simulink model "sensor_vehicle_modell"  (R2021a)
settings: Solver=ode3  StartTime=0.0  StopTime=70  FixedStep=0.01  RelTol=1e-3
values from neighbouring files (symbols this model uses):
  A = 2    [Parameter.m]
  cw = 0.0    (= 0)    [Parameter.m]
  d = 0.63    [Parameter.m]
  m = 1500    [Parameter.m]
  p = 1.2    [Parameter.m]
undefined symbols (not defined in the file or in its folder): DiscIntNeverNeededParam
libraries: simulink x4, simulink_extras x1
settings Model: Creator=ge78kon  LastModifiedBy=admin
settings SolverCC: AlgebraicLoopSolver=TrustRegion
settings DataIOCC: ReturnWorkspaceOutputs=off
settings DebuggingCC: SFMachineParentedDataDiag=warning  ArithmeticOperatorsInVariantConditions=warning
settings SFSimCC: CustomCodeUndefinedFunction=UseInterfaceOnly

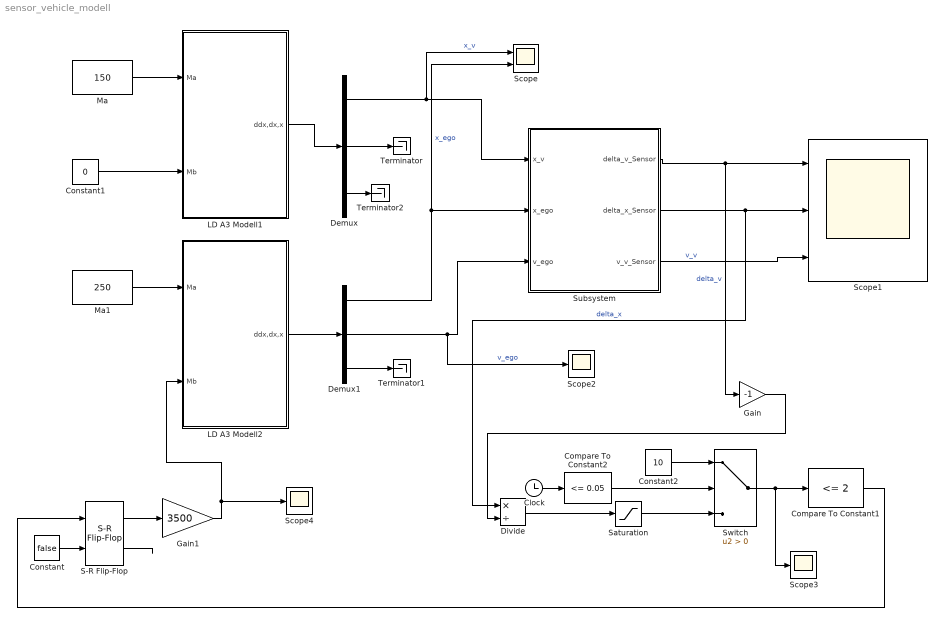
== system sensor_vehicle_modell ==
  Clock : Clock
  Compare To Constant1 : simulink/Logic and Bit Operations/Compare To Constant  relop=<=  const=2  OutDataTypeStr=boolean
  Compare To Constant2 : simulink/Logic and Bit Operations/Compare To Constant  relop=<=  const=0.05  OutDataTypeStr=boolean
  Constant : Constant  Value=false
  Constant1 : Constant  Value=0
  Constant2 : Constant  Value=10
  Demux : Demux  Outputs=3
  Demux1 : Demux  Outputs=3
  Divide : Product  Inputs=*/
  Gain : Gain  Gain=-1
  Gain1 : Gain  Gain=3500
  LD A3 Modell1 : Subsystem  mask{x_start=450, v_start=20}
      mask prompts: x_start "Startposition"; v_start "Startgeschwindigkeit"
  LD A3 Modell2 : Subsystem  mask{x_start=0, v_start=30}
      mask prompts: x_start "Startposition"; v_start "Startgeschwindigkeit"
  Ma : Constant  Value=150
  Ma1 : Constant  Value=250
  S-R Flip-Flop : simulink_extras/Flip Flops/S-R Flip-Flop  initial_condition=0
  Saturation : Saturate  UpperLimit=10
  Scope : Scope  NumInputPorts=2
  Scope1 : Scope  NumInputPorts=3
  Scope2 : Scope
  Scope3 : Scope
  Scope4 : Scope
  Subsystem : Subsystem  mask{Rauschen=off}
      mask prompts: Rauschen "Rauschen an/aus"
  Switch : Switch  Criteria=u2 > Threshold
  Terminator : Terminator
  Terminator1 : Terminator
  Terminator2 : Terminator
  wires:
  Ma/1 -> LD A3 Modell1/1("Ma ")
  Constant1/1 -> LD A3 Modell1/2("Mb ")
  LD A3 Modell1/1(ddx,dx,x) -> Demux/1
  LD A3 Modell2/1(ddx,dx,x) -> Demux1/1
  Ma1/1 -> LD A3 Modell2/1("Ma ")
  Demux/2 -> Terminator/1
  Demux1/3 -> Terminator1/1
  Demux/1 -> Scope/1, Subsystem/1(x_v)  "x_v"
  Demux1/1 -> Scope/2, Subsystem/2(x_ego)  "x_ego"
  Demux1/2 -> Scope2/1, Subsystem/3(v_ego)  "v_ego"
  Subsystem/1(delta_v_Sensor) -> Scope1/1, Gain/1  "delta_v"
  Subsystem/2(delta_x_Sensor) -> Divide/1, Scope1/2  "delta_x"
  Subsystem/3(v_v_Sensor) -> Scope1/3  "v_v"
  Demux/3 -> Terminator2/1
  Gain/1 -> Divide/2
  Divide/1 -> Saturation/1
  Compare To Constant1/1 -> S-R Flip-Flop/1
  S-R Flip-Flop/1 -> Gain1/1
  Gain1/1 -> LD A3 Modell2/2("Mb "), Scope4/1
  Constant/1 -> S-R Flip-Flop/2
  Clock/1 -> Compare To Constant2/1
  Compare To Constant2/1 -> Switch/2
  Constant2/1 -> Switch/1
  Saturation/1 -> Switch/3
  Switch/1 -> Scope3/1, Compare To Constant1/1
  S-R Flip-Flop/2 -> ?

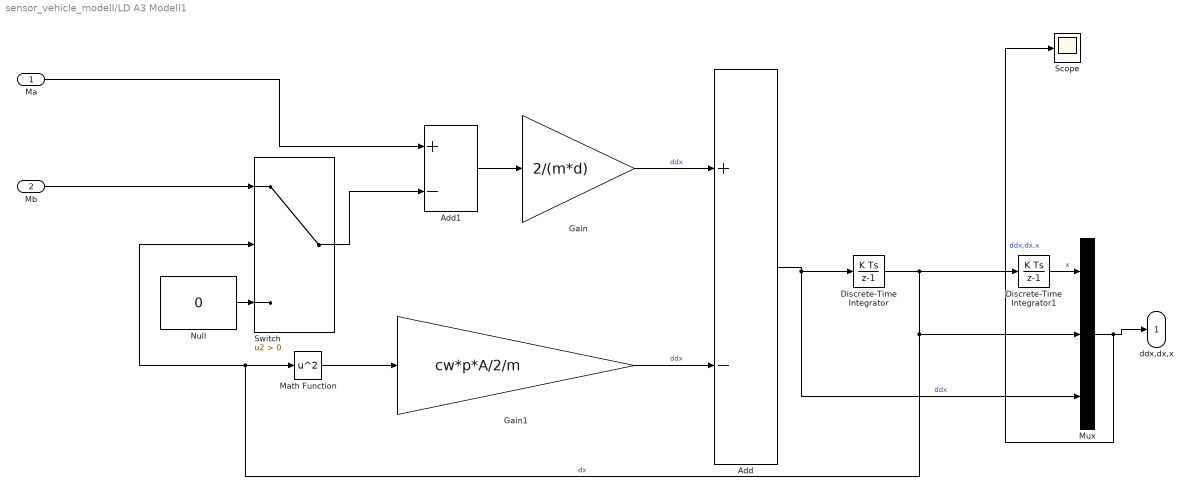
== system sensor_vehicle_modell/LD A3 Modell1 ==
  "Ma " : Inport
  "Mb " : Inport  Port=2
  Add : Sum  Inputs=+-
  Add1 : Sum  Inputs=+-
  Discrete-Time Integrator : DiscreteIntegrator  InitialCondition=v_start  SampleTime=-1  ICPrevOutput=DiscIntNeverNeededParam  ICPrevScaledInput=DiscIntNeverNeededParam
  Discrete-Time Integrator1 : DiscreteIntegrator  InitialCondition=x_start  SampleTime=-1  ICPrevOutput=DiscIntNeverNeededParam  ICPrevScaledInput=DiscIntNeverNeededParam
  Gain : Gain  Gain=2/(m*d)
  Gain1 : Gain  Gain=cw*p*A/2/m
  Math Function : Math  Operator=square  SignedPower=on  SaturateOnIntegerOverflow=on
  Mux : Mux  Inputs=3
  Null : Constant  Value=0
  Scope : Scope
  Switch : Switch  Criteria=u2 > Threshold
  ddx,dx,x : Outport  VectorParamsAs1DForOutWhenUnconnected=off
  wires:
  "Ma "/1 -> Add1/1
  Add1/1 -> Gain/1
  Discrete-Time Integrator/1 -> Switch/2, Math Function/1, Mux/2, Discrete-Time Integrator1/1  "dx"
  Gain1/1 -> Add/2  "ddx"
  Gain/1 -> Add/1  "ddx"
  Null/1 -> Switch/3
  Add/1 -> Discrete-Time Integrator/1, Mux/3  "ddx"
  Math Function/1 -> Gain1/1
  Switch/1 -> Add1/2
  Discrete-Time Integrator1/1 -> Mux/1  "x"
  "Mb "/1 -> Switch/1
  Mux/1 -> Scope/1, ddx,dx,x/1  "ddx,dx,x"

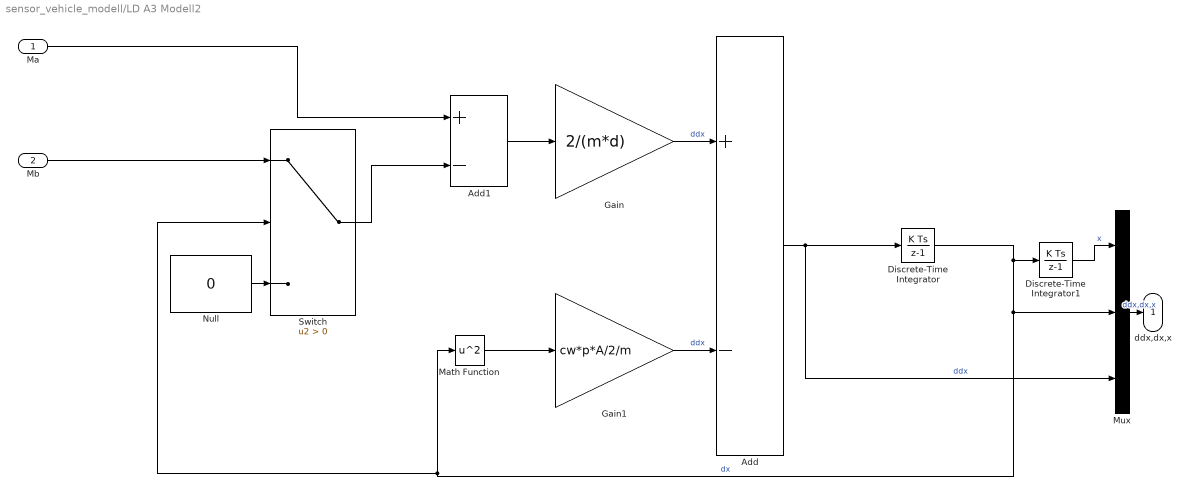
== system sensor_vehicle_modell/LD A3 Modell2 ==
  "Ma " : Inport
  "Mb " : Inport  Port=2
  Add : Sum  Inputs=+-
  Add1 : Sum  Inputs=+-
  Discrete-Time Integrator : DiscreteIntegrator  InitialCondition=v_start  SampleTime=-1  ICPrevOutput=DiscIntNeverNeededParam  ICPrevScaledInput=DiscIntNeverNeededParam
  Discrete-Time Integrator1 : DiscreteIntegrator  InitialCondition=x_start  SampleTime=-1  ICPrevOutput=DiscIntNeverNeededParam  ICPrevScaledInput=DiscIntNeverNeededParam
  Gain : Gain  Gain=2/(m*d)
  Gain1 : Gain  Gain=cw*p*A/2/m
  Math Function : Math  Operator=square  SignedPower=on  SaturateOnIntegerOverflow=on
  Mux : Mux  Inputs=3
  Null : Constant  Value=0
  Switch : Switch  Criteria=u2 > Threshold
  ddx,dx,x : Outport  VectorParamsAs1DForOutWhenUnconnected=off
  wires:
  "Ma "/1 -> Add1/1
  Add1/1 -> Gain/1
  Discrete-Time Integrator/1 -> Mux/2, Switch/2, Math Function/1, Discrete-Time Integrator1/1  "dx"
  Gain1/1 -> Add/2  "ddx"
  Gain/1 -> Add/1  "ddx"
  Null/1 -> Switch/3
  Add/1 -> Discrete-Time Integrator/1, Mux/3  "ddx"
  Math Function/1 -> Gain1/1
  Switch/1 -> Add1/2
  Discrete-Time Integrator1/1 -> Mux/1  "x"
  "Mb "/1 -> Switch/1
  Mux/1 -> ddx,dx,x/1  "ddx,dx,x"

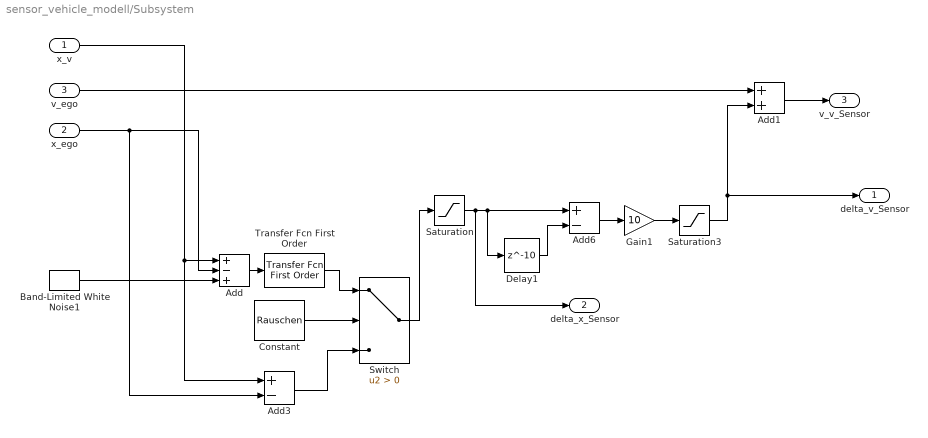
== system sensor_vehicle_modell/Subsystem ==
  x_v : Inport
  x_ego : Inport  Port=2
  v_ego : Inport  Port=3
  Add : Sum  Inputs=+-+
  Add1 : Sum
  Add3 : Sum  Inputs=+-
  Add6 : Sum  Inputs=+-
  Band-Limited White Noise1 : simulink/Sources/Band-Limited White Noise  Cov=[0.007]  Ts=0.01  seed=[23341]
  Constant : Constant  Value=Rauschen
  Delay1 : Delay  DelayLength=10
  Gain1 : Gain  Gain=10
  Saturation : Saturate  UpperLimit=200  LowerLimit=0
  Saturation3 : Saturate  UpperLimit=-0.01  LowerLimit=-50
  Switch : Switch  Criteria=u2 > Threshold
  Transfer Fcn First Order : simulink/Discrete/Transfer Fcn First Order  PoleZ=0.99  ICPrevOutput=0.0  DoSatur=off
  delta_v_Sensor : Outport  VectorParamsAs1DForOutWhenUnconnected=off
  delta_x_Sensor : Outport  Port=2  VectorParamsAs1DForOutWhenUnconnected=off
  v_v_Sensor : Outport  Port=3  VectorParamsAs1DForOutWhenUnconnected=off
  wires:
  Saturation/1 -> delta_x_Sensor/1, Delay1/1, Add6/1
  Add6/1 -> Gain1/1
  x_ego/1 -> Add3/2, Add/2
  x_v/1 -> Add/1, Add3/1
  Band-Limited White Noise1/1 -> Add/3
  Delay1/1 -> Add6/2
  Switch/1 -> Saturation/1
  v_ego/1 -> Add1/1
  Saturation3/1 -> delta_v_Sensor/1, Add1/2
  Gain1/1 -> Saturation3/1
  Add1/1 -> v_v_Sensor/1
  Constant/1 -> Switch/2
  Add3/1 -> Switch/3
  Add/1 -> Transfer Fcn First Order/1
  Transfer Fcn First Order/1 -> Switch/1
